simulink library "sixDoFDynamics_ul"  (R2018b)
settings: Solver=VariableStepAuto  StartTime=0.0  StopTime=10.0  RelTol=1e-3
libraries: vrlib x2, simulink x1, eulAng2RotMat_ul x1, eulDot x1
settings Model: Creator=mcobb  LastModifiedBy=asiddiq2

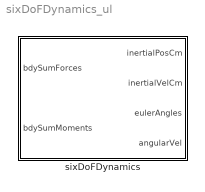
== system sixDoFDynamics_ul ==
  sixDoFDynamics : Subsystem  mask{massBdy=10, massAdded=zeros(3,3), bdy_MI_cm=eye(3), initPosCM=[0;0;100], initVelCM=[0;0;0], initEulAngs=[0;0;0], initAngVel=[0;0;0]}
      mask prompts: massBdy "Mass"; massAdded "Added Mass Matrix"; bdy_MI_cm "Inertia matrix"; initPosCM "Initial position"; initVelCM "Initial velocity"; initEulAngs "Initial Euler Angles"; initAngVel "Initial Angular Velocity"
      mask init:
      | Mtot_inverse = inv(massBdy*eye(3) + massAdded);
      | bdy_MI_inv = inv(bdy_MI_cm);
      mask DialogControl ParameterGroupVar Prompt: Vehicle
      mask DialogControl Container3 Prompt: Initial conditions

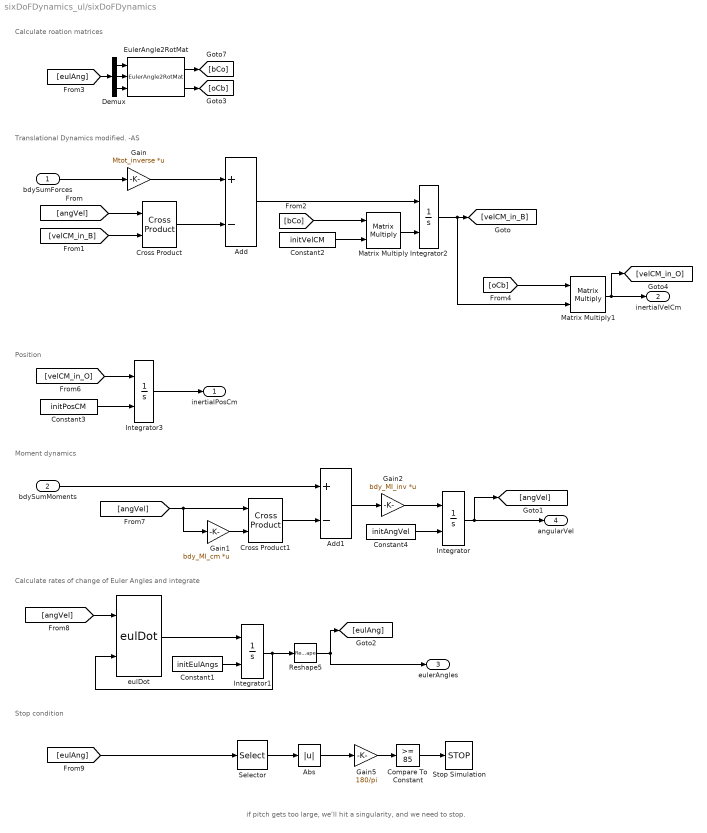
== system sixDoFDynamics_ul/sixDoFDynamics ==
  note: Position
  note: Calculate roation matrices
  note: Stop condition
  note: Moment dynamics
  note: Calculate rates of change of Euler Angles and integrate
  note: Translational Dynamics modified. -AS
  note: if pitch gets too large, we'll hit a singularity, and we need to stop.
  bdySumForces : Inport  PortDimensions=[3,1]
  bdySumMoments : Inport  Port=2  PortDimensions=[3,1]
  Abs : Abs
  Add : Sum  Inputs=+-
  Add1 : Sum  Inputs=+-
  Compare To Constant : simulink/Logic and Bit Operations/Compare To Constant  relop=>=  const=85  OutDataTypeStr=boolean
  Constant1 : Constant  Value=initEulAngs  VectorParams1D=off
  Constant2 : Constant  Value=initVelCM  VectorParams1D=off
  Constant3 : Constant  Value=initPosCM  VectorParams1D=off
  Constant4 : Constant  Value=initAngVel  VectorParams1D=off
  Cross Product : vrlib/Utilities/Cross Product
      settings: SourceProductBaseCode=VR
  Cross Product1 : vrlib/Utilities/Cross Product
      settings: SourceProductBaseCode=VR
  Demux : Demux  Outputs=3
  EulerAngle2RotMat : eulAng2RotMat_ul/EulerAngle2RotMat  SystemSampleTime=-1
  Gain : Gain  Gain=Mtot_inverse  Multiplication=Matrix(K*u)
  Gain1 : Gain  Gain=bdy_MI_cm  Multiplication=Matrix(K*u)
  Gain2 : Gain  Gain=bdy_MI_inv  Multiplication=Matrix(K*u)
  Gain5 : Gain  Gain=180/pi
  Integrator : Integrator  InitialConditionSource=external
  Integrator1 : Integrator  InitialConditionSource=external  InitialCondition=initEulAngs
  Integrator2 : Integrator  InitialConditionSource=external
  Integrator3 : Integrator  InitialConditionSource=external
  Matrix Multiply : Product  Multiplication=Matrix(*)
  Matrix Multiply1 : Product  Multiplication=Matrix(*)
  Reshape5 : Reshape  OutputDimensionality=Column vector (2-D)
  Selector : Selector  InputPortWidth=3  IndexOptions=Index vector (dialog)  Indices=2  OutputSizes=1
  Stop Simulation : Stop
  eulDot : eulDot/eulDot  SystemSampleTime=-1
  inertialPosCm : Outport
  inertialVelCm : Outport  Port=2
  eulerAngles : Outport  Port=3  PortDimensions=[3,1]
  angularVel : Outport  Port=4  PortDimensions=[3,1]
  wires:
  Compare To Constant/1 -> Stop Simulation/1
  Gain5/1 -> Compare To Constant/1
  Abs/1 -> Gain5/1
  Selector/1 -> Abs/1
  EulerAngle2RotMat/2 -> [oCb]
  EulerAngle2RotMat/1 -> [bCo]
  Demux/3 -> EulerAngle2RotMat/3
  Demux/2 -> EulerAngle2RotMat/2
  Demux/1 -> EulerAngle2RotMat/1
  [eulAng] -> Demux/1
  Reshape5/1 -> eulerAngles/1, [eulAng]
  Constant1/1 -> Integrator1/2
  eulDot/1 -> Integrator1/1
  bdySumForces/1 -> Gain/1
  Integrator1/1 -> Reshape5/1, eulDot/2
  Gain/1 -> Add/1
  Cross Product/1 -> Add/2
  [angVel] -> Cross Product/1
  [velCM_in_B] -> Cross Product/2
  Add/1 -> Integrator2/1
  Constant2/1 -> Matrix Multiply/2
  [bCo] -> Matrix Multiply/1
  Matrix Multiply/1 -> Integrator2/2
  [oCb] -> Matrix Multiply1/1
  Matrix Multiply1/1 -> [velCM_in_O], inertialVelCm/1
  Integrator2/1 -> Matrix Multiply1/2, [velCM_in_B]
  [velCM_in_O] -> Integrator3/1
  Constant3/1 -> Integrator3/2
  Integrator3/1 -> inertialPosCm/1
  bdySumMoments/1 -> Add1/1
  [angVel] -> Gain1/1, Cross Product1/1
  Gain1/1 -> Cross Product1/2
  Cross Product1/1 -> Add1/2
  Add1/1 -> Gain2/1
  Integrator/1 -> angularVel/1, [angVel]
  [angVel] -> eulDot/1
  [eulAng] -> Selector/1
  Gain2/1 -> Integrator/1
  Constant4/1 -> Integrator/2
